simulink model "test_kinematics_sim"  (R2021b)
settings: Solver=ode8  StartTime=0.0  StopTime=100  FixedStep=0.01  RelTol=1e-3
values from neighbouring files (symbols this model uses):
  A = A0t'    [test_kinematics.m]
  e_angles0 = [atan(-A(2,1)/A(2,2)),asin(A(2,3)),atan(-A(1,3)/A(3,3))]    [test_kinematics.m]
  h0 = [Ix*omega0(1) Iy*omega0(2) Iz*omega0(3)]'    [test_kinematics.m]
  invJ = inv(J)    [test_kinematics.m]
  J = [Ix 0 0; 0 Iy 0; 0 0 Iz]    [test_kinematics.m]
  omega0 = [C 0.1 0.1]    [test_kinematics.m]
libraries: kinematic_transform x1, kinematics x1
settings Model: Creator=Davide  LastModifiedBy=Davide

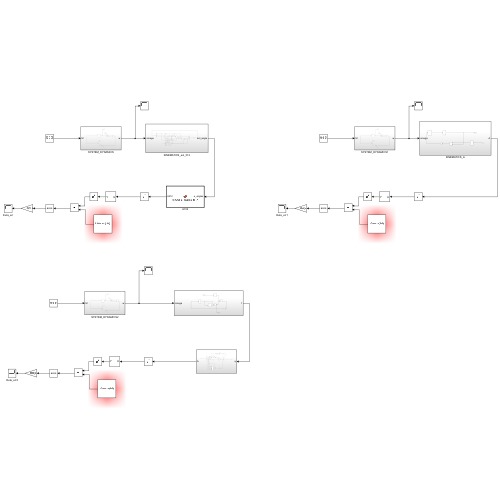
[thumbnail: Simulink's stored preview of the top-level diagram]
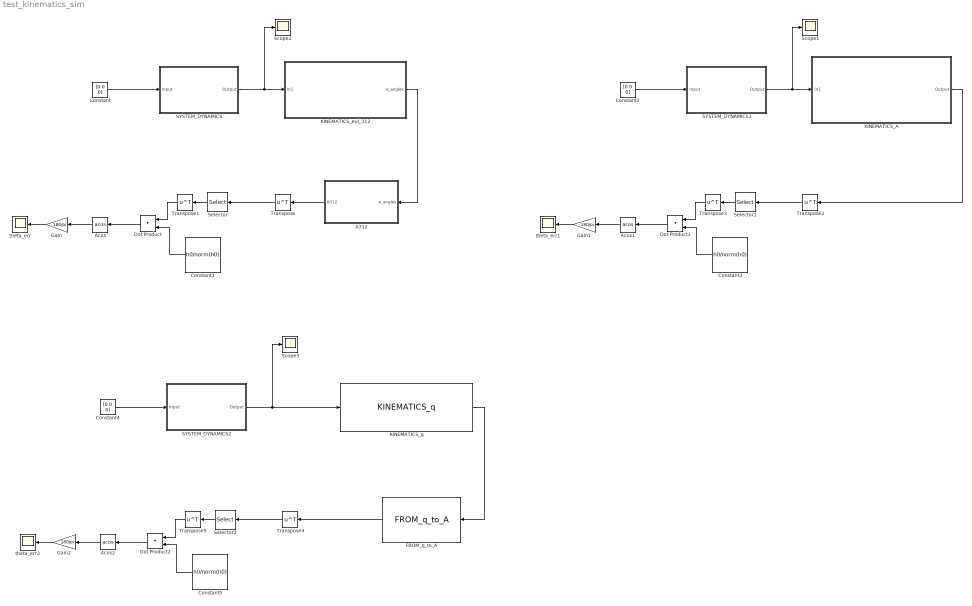
== system test_kinematics_sim ==
  A312 : MATLAB Function  TreatAsAtomicUnit=on
  Acos : Trigonometry  Operator=acos
  Acos1 : Trigonometry  Operator=acos
  Acos2 : Trigonometry  Operator=acos
  Constant : Constant  Value=[0 0 0]
  Constant1 : Constant  Value=h0/norm(h0)
  Constant2 : Constant  Value=[0 0 0]
  Constant3 : Constant  Value=h0/norm(h0)
  Constant4 : Constant  Value=[0 0 0]
  Constant5 : Constant  Value=h0/norm(h0)
  Dot Product : DotProduct  InputSameDT=on  OutDataTypeStr=Inherit: Inherit via internal rule
  Dot Product1 : DotProduct  InputSameDT=on  OutDataTypeStr=Inherit: Inherit via internal rule
  Dot Product2 : DotProduct  InputSameDT=on  OutDataTypeStr=Inherit: Inherit via internal rule
  FROM_q_to_A : kinematic_transform/FROM_q_to_A  SystemSampleTime=-1  VariantActivationTime=update diagram  Latency=0  AutoFrameSizeCalculation=off
      settings: SourceProductName=Kinematic Tranformation
  Gain : Gain  Gain=180/pi
  Gain1 : Gain  Gain=180/pi
  Gain2 : Gain  Gain=180/pi
  KINEMATICS_A : Subsystem
  KINEMATICS_eul_312 : Subsystem
  KINEMATICS_q : kinematics/KINEMATICS_q  SystemSampleTime=-1  VariantActivationTime=update diagram  Latency=0  AutoFrameSizeCalculation=off
  SYSTEM_DYNAMICS : Subsystem
  SYSTEM_DYNAMICS1 : Subsystem
  SYSTEM_DYNAMICS2 : Subsystem
  Scope1 : Scope
  Scope2 : Scope
  Scope3 : Scope
  Selector : Selector  NumberOfDimensions=2  InputPortWidth=3  IndexOptions=Index vector (dialog),Select all  Indices=1,1  OutputSizes=1,1
  Selector1 : Selector  NumberOfDimensions=2  InputPortWidth=3  IndexOptions=Index vector (dialog),Select all  Indices=1,1  OutputSizes=1,1
  Selector2 : Selector  NumberOfDimensions=2  InputPortWidth=3  IndexOptions=Index vector (dialog),Select all  Indices=1,1  OutputSizes=1,1
  Transpose{,1..5} (6 alike) : Math  Operator=transpose  SaturateOnIntegerOverflow=on
  theta_err : Scope
  theta_err1 : Scope
  theta_err2 : Scope
  wires:
  Constant/1 -> SYSTEM_DYNAMICS/1(Input)
  SYSTEM_DYNAMICS/1(Output) -> KINEMATICS_eul_312/1(In1), Scope2/1
  A312/1(A312) -> Transpose/1
  Selector/1 -> Transpose1/1
  Constant1/1 -> Dot Product/2
  Dot Product/1 -> Acos/1
  Acos/1 -> Gain/1
  Gain/1 -> theta_err/1
  Transpose1/1 -> Dot Product/1
  KINEMATICS_eul_312/1(e_angles) -> A312/1(e_angles)
  Transpose/1 -> Selector/1
  KINEMATICS_A/1(Output) -> Transpose2/1
  Gain1/1 -> theta_err1/1
  Transpose3/1 -> Dot Product1/1
  Selector1/1 -> Transpose3/1
  SYSTEM_DYNAMICS1/1(Output) -> KINEMATICS_A/1(In1), Scope1/1
  Acos1/1 -> Gain1/1
  Transpose2/1 -> Selector1/1
  Constant3/1 -> Dot Product1/2
  Dot Product1/1 -> Acos1/1
  Constant2/1 -> SYSTEM_DYNAMICS1/1(Input)
  Dot Product2/1 -> Acos2/1
  SYSTEM_DYNAMICS2/1(Output) -> Scope3/1, KINEMATICS_q/1
  Acos2/1 -> Gain2/1
  Constant4/1 -> SYSTEM_DYNAMICS2/1(Input)
  Selector2/1 -> Transpose5/1
  Transpose5/1 -> Dot Product2/1
  Gain2/1 -> theta_err2/1
  Transpose4/1 -> Selector2/1
  Constant5/1 -> Dot Product2/2
  FROM_q_to_A/1 -> Transpose4/1
  KINEMATICS_q/1 -> FROM_q_to_A/1

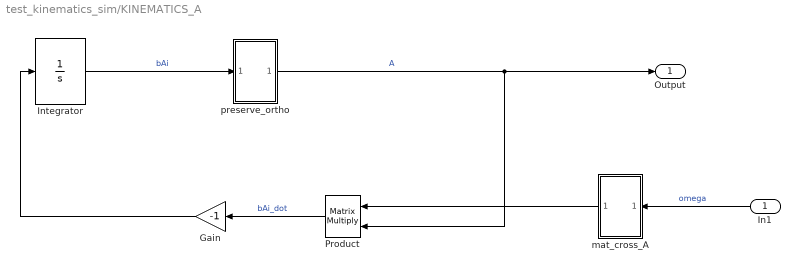
== system test_kinematics_sim/KINEMATICS_A ==
  In1 : Inport
  Gain : Gain  Gain=-1
  Integrator : Integrator  InitialCondition=A
  Product : Product  Multiplication=Matrix(*)
  mat_cross_A : Subsystem
  preserve_ortho : Subsystem
  Output : Outport
  wires:
  Integrator/1 -> preserve_ortho/1(In1)  "bAi"
  Product/1 -> Gain/1  "bAi_dot"
  In1/1 -> mat_cross_A/1(In1)  "omega"
  preserve_ortho/1(Out1) -> Output/1, Product/2  "A"
  mat_cross_A/1(Out1) -> Product/1
  Gain/1 -> Integrator/1

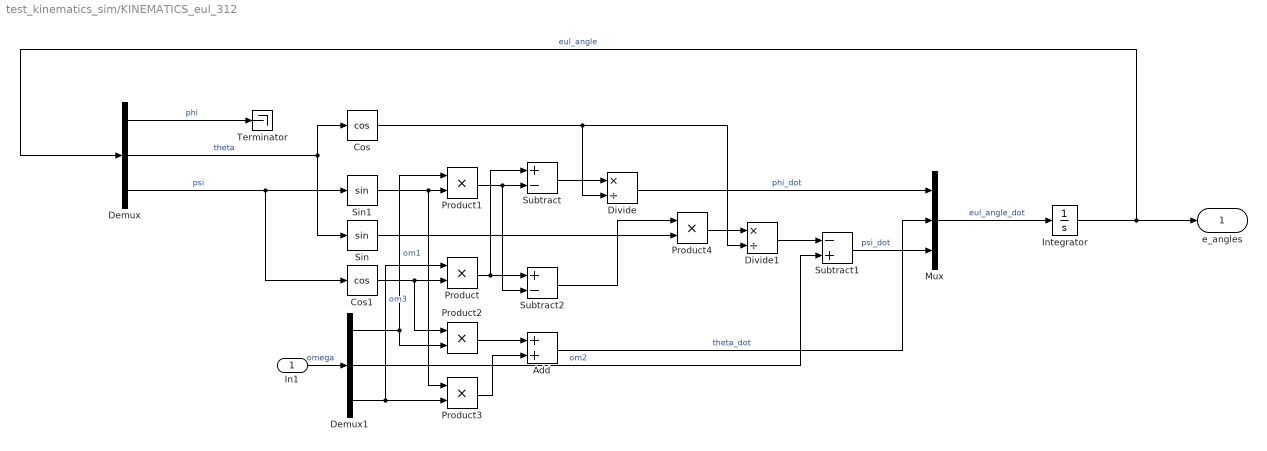
== system test_kinematics_sim/KINEMATICS_eul_312 ==
  In1 : Inport
  Add : Sum
  Cos : Trigonometry  Operator=cos
  Cos1 : Trigonometry  Operator=cos
  Demux : Demux  Outputs=3
  Demux1 : Demux  Outputs=3
  Divide : Product  Inputs=*/
  Divide1 : Product  Inputs=*/
  Integrator : Integrator  InitialCondition=e_angles0
  Mux : Mux  Inputs=3
  Product{,1..4} (5 alike) : Product
  Sin : Trigonometry
  Sin1 : Trigonometry
  Subtract : Sum  Inputs=+-
  Subtract1 : Sum  Inputs=-+
  Subtract2 : Sum  Inputs=+-
  Terminator : Terminator
  e_angles : Outport
  wires:
  Add/1 -> Mux/2  "theta_dot"
  In1/1 -> Demux1/1  "omega"
  Product2/1 -> Add/1
  Cos/1 -> Divide1/2, Divide/2
  Product3/1 -> Add/2
  Divide/1 -> Mux/1  "phi_dot"
  Demux/1 -> Terminator/1  "phi"
  Integrator/1 -> Demux/1, e_angles/1  "eul_angle"
  Cos1/1 -> Product2/1, Product/2
  Sin/1 -> Product4/2
  Product1/1 -> Subtract2/2, Subtract/2
  Divide1/1 -> Subtract1/1
  Demux/3 -> Sin1/1, Cos1/1  "psi"
  Subtract/1 -> Divide/1
  Demux1/3 -> Product3/2, Product/1  "om3"
  Mux/1 -> Integrator/1  "eul_angle_dot"
  Product/1 -> Subtract2/1, Subtract/1
  Product4/1 -> Divide1/1
  Demux1/1 -> Product2/2, Product1/1  "om1"
  Demux/2 -> Cos/1, Sin/1  "theta"
  Sin1/1 -> Product3/1, Product1/2
  Subtract2/1 -> Product4/1
  Demux1/2 -> Subtract1/2  "om2"
  Subtract1/1 -> Mux/3  "psi_dot"

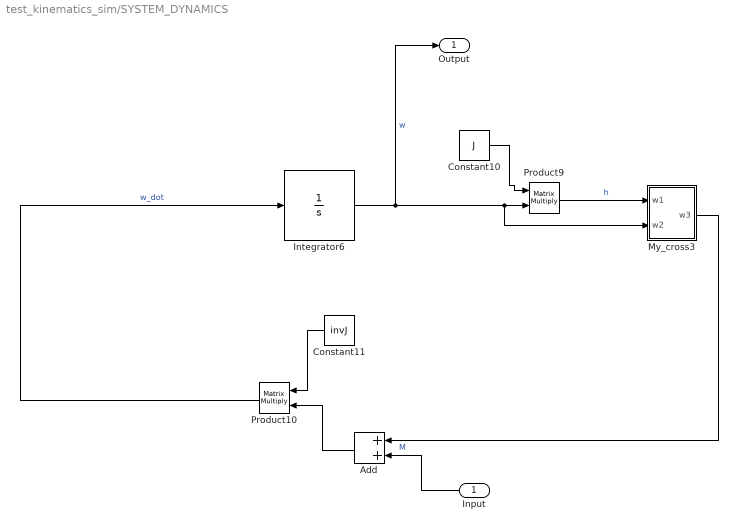
== system test_kinematics_sim/SYSTEM_DYNAMICS ==
  Input : Inport
  Add : Sum
  Constant10 : Constant  Value=J
  Constant11 : Constant  Value=invJ
  Integrator6 : Integrator  InitialCondition=omega0
  My_cross3 : Subsystem
  Product10 : Product  Multiplication=Matrix(*)
  Product9 : Product  Multiplication=Matrix(*)
  Output : Outport
  wires:
  Integrator6/1 -> Output/1, My_cross3/2(w2), Product9/2  "w"
  Constant10/1 -> Product9/1
  Constant11/1 -> Product10/1
  Product9/1 -> My_cross3/1(w1)  "h"
  My_cross3/1(w3) -> Add/1
  Product10/1 -> Integrator6/1  "w_dot"
  Input/1 -> Add/2  "M"
  Add/1 -> Product10/2

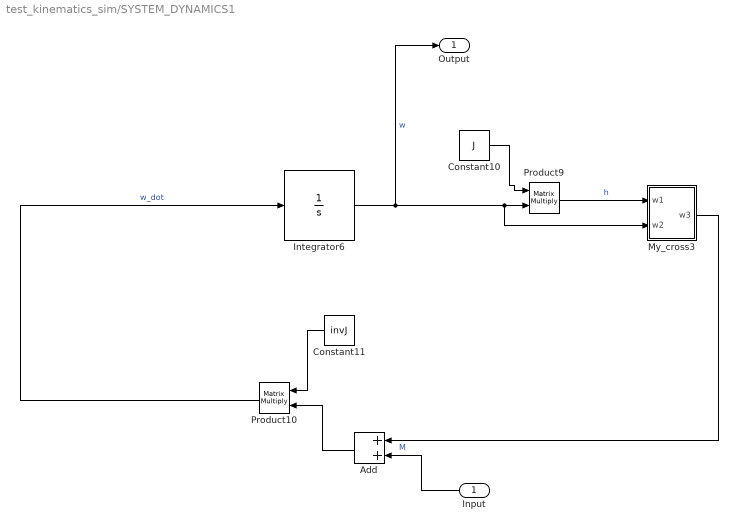
== system test_kinematics_sim/SYSTEM_DYNAMICS1 ==
  Input : Inport
  Add : Sum
  Constant10 : Constant  Value=J
  Constant11 : Constant  Value=invJ
  Integrator6 : Integrator  InitialCondition=omega0
  My_cross3 : Subsystem
  Product10 : Product  Multiplication=Matrix(*)
  Product9 : Product  Multiplication=Matrix(*)
  Output : Outport
  wires:
  Integrator6/1 -> Output/1, My_cross3/2(w2), Product9/2  "w"
  Constant10/1 -> Product9/1
  Constant11/1 -> Product10/1
  Product9/1 -> My_cross3/1(w1)  "h"
  My_cross3/1(w3) -> Add/1
  Product10/1 -> Integrator6/1  "w_dot"
  Input/1 -> Add/2  "M"
  Add/1 -> Product10/2

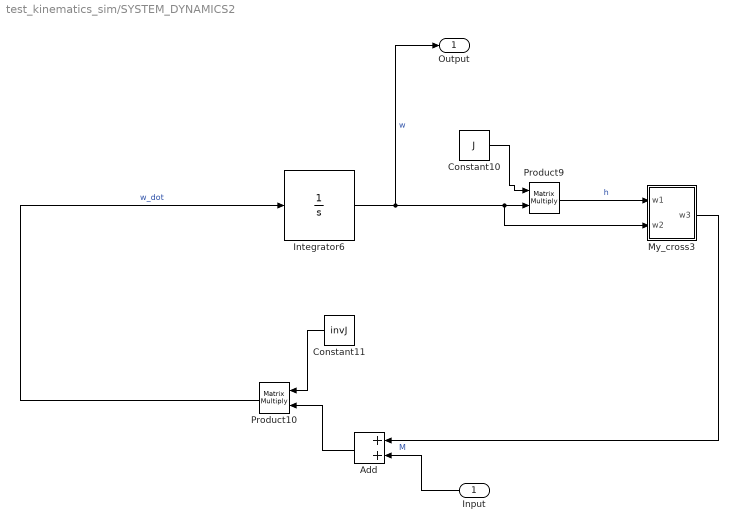
== system test_kinematics_sim/SYSTEM_DYNAMICS2 ==
  Input : Inport
  Add : Sum
  Constant10 : Constant  Value=J
  Constant11 : Constant  Value=invJ
  Integrator6 : Integrator  InitialCondition=omega0
  My_cross3 : Subsystem
  Product10 : Product  Multiplication=Matrix(*)
  Product9 : Product  Multiplication=Matrix(*)
  Output : Outport
  wires:
  Integrator6/1 -> Output/1, My_cross3/2(w2), Product9/2  "w"
  Constant10/1 -> Product9/1
  Constant11/1 -> Product10/1
  Product9/1 -> My_cross3/1(w1)  "h"
  My_cross3/1(w3) -> Add/1
  Product10/1 -> Integrator6/1  "w_dot"
  Input/1 -> Add/2  "M"
  Add/1 -> Product10/2

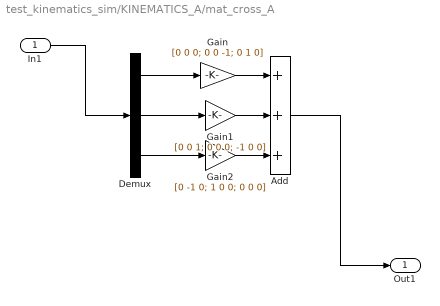
== system test_kinematics_sim/KINEMATICS_A/mat_cross_A ==
  In1 : Inport
  Add : Sum  Inputs=+++
  Demux : Demux  Outputs=3
  Gain : Gain  Gain=[0 0 0; 0 0 -1; 0 1 0]
  Gain1 : Gain  Gain=[0 0 1; 0 0 0; -1 0 0]
  Gain2 : Gain  Gain=[0 -1 0; 1 0 0; 0 0 0]
  Out1 : Outport
  wires:
  In1/1 -> Demux/1
  Gain1/1 -> Add/2
  Gain2/1 -> Add/3
  Demux/2 -> Gain1/1
  Add/1 -> Out1/1
  Gain/1 -> Add/1
  Demux/3 -> Gain2/1
  Demux/1 -> Gain/1

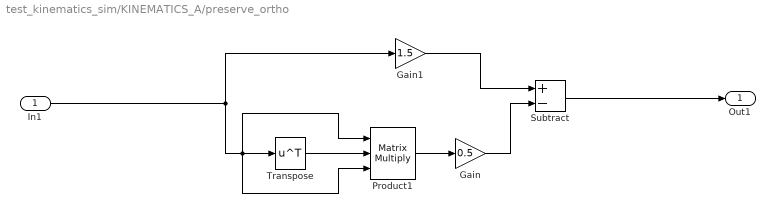
== system test_kinematics_sim/KINEMATICS_A/preserve_ortho ==
  In1 : Inport
  Gain : Gain  Gain=0.5
  Gain1 : Gain  Gain=1.5
  Product1 : Product  Inputs=3  Multiplication=Matrix(*)
  Subtract : Sum  Inputs=+-
  Transpose : Math  Operator=transpose  SaturateOnIntegerOverflow=on
  Out1 : Outport
  wires:
  In1/1 -> Product1/3, Product1/1, Transpose/1, Gain1/1
  Gain1/1 -> Subtract/1
  Product1/1 -> Gain/1
  Gain/1 -> Subtract/2
  Transpose/1 -> Product1/2
  Subtract/1 -> Out1/1

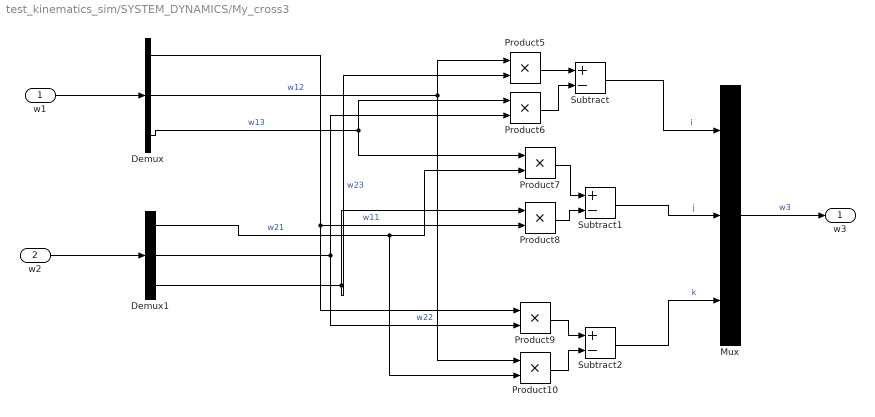
== system test_kinematics_sim/SYSTEM_DYNAMICS/My_cross3 ==
  w1 : Inport
  w2 : Inport  Port=2
  Demux : Demux  Outputs=3
  Demux1 : Demux  Outputs=3
  Mux : Mux  Inputs=3
  Product{5..10} (6 alike) : Product
  Subtract : Sum  Inputs=+-
  Subtract1 : Sum  Inputs=+-
  Subtract2 : Sum  Inputs=+-
  w3 : Outport
  wires:
  Subtract1/1 -> Mux/2  "j"
  Product6/1 -> Subtract/2
  Demux1/3 -> Product5/2, Product8/1  "w23"
  Demux/1 -> Product9/1, Product8/2  "w11"
  Demux/3 -> Product7/1, Product6/1  "w13"
  Product5/1 -> Subtract/1
  Demux1/1 -> Product10/2, Product7/2  "w21"
  Product9/1 -> Subtract2/1
  Demux1/2 -> Product9/2, Product6/2  "w22"
  Demux/2 -> Product5/1, Product10/1  "w12"
  Subtract/1 -> Mux/1  "i"
  w2/1 -> Demux1/1
  Product10/1 -> Subtract2/2
  Product7/1 -> Subtract1/1
  Product8/1 -> Subtract1/2
  Subtract2/1 -> Mux/3  "k"
  w1/1 -> Demux/1
  Mux/1 -> w3/1  "w3"

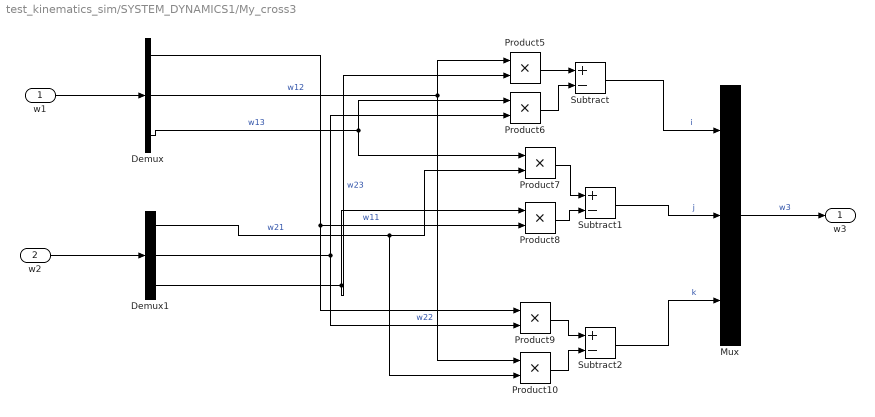
== system test_kinematics_sim/SYSTEM_DYNAMICS1/My_cross3 ==
  w1 : Inport
  w2 : Inport  Port=2
  Demux : Demux  Outputs=3
  Demux1 : Demux  Outputs=3
  Mux : Mux  Inputs=3
  Product{5..10} (6 alike) : Product
  Subtract : Sum  Inputs=+-
  Subtract1 : Sum  Inputs=+-
  Subtract2 : Sum  Inputs=+-
  w3 : Outport
  wires:
  Subtract1/1 -> Mux/2  "j"
  Product6/1 -> Subtract/2
  Demux1/3 -> Product5/2, Product8/1  "w23"
  Demux/1 -> Product9/1, Product8/2  "w11"
  Demux/3 -> Product7/1, Product6/1  "w13"
  Product5/1 -> Subtract/1
  Demux1/1 -> Product10/2, Product7/2  "w21"
  Product9/1 -> Subtract2/1
  Demux1/2 -> Product9/2, Product6/2  "w22"
  Demux/2 -> Product5/1, Product10/1  "w12"
  Subtract/1 -> Mux/1  "i"
  w2/1 -> Demux1/1
  Product10/1 -> Subtract2/2
  Product7/1 -> Subtract1/1
  Product8/1 -> Subtract1/2
  Subtract2/1 -> Mux/3  "k"
  w1/1 -> Demux/1
  Mux/1 -> w3/1  "w3"

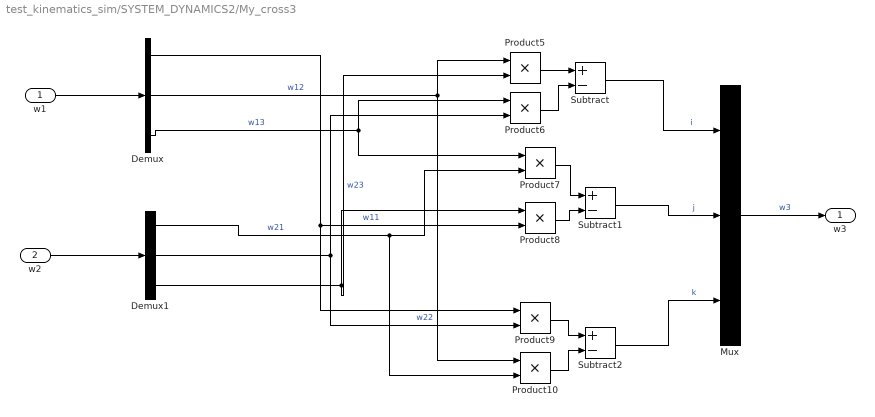
== system test_kinematics_sim/SYSTEM_DYNAMICS2/My_cross3 ==
  w1 : Inport
  w2 : Inport  Port=2
  Demux : Demux  Outputs=3
  Demux1 : Demux  Outputs=3
  Mux : Mux  Inputs=3
  Product{5..10} (6 alike) : Product
  Subtract : Sum  Inputs=+-
  Subtract1 : Sum  Inputs=+-
  Subtract2 : Sum  Inputs=+-
  w3 : Outport
  wires:
  Subtract1/1 -> Mux/2  "j"
  Product6/1 -> Subtract/2
  Demux1/3 -> Product5/2, Product8/1  "w23"
  Demux/1 -> Product9/1, Product8/2  "w11"
  Demux/3 -> Product7/1, Product6/1  "w13"
  Product5/1 -> Subtract/1
  Demux1/1 -> Product10/2, Product7/2  "w21"
  Product9/1 -> Subtract2/1
  Demux1/2 -> Product9/2, Product6/2  "w22"
  Demux/2 -> Product5/1, Product10/1  "w12"
  Subtract/1 -> Mux/1  "i"
  w2/1 -> Demux1/1
  Product10/1 -> Subtract2/2
  Product7/1 -> Subtract1/1
  Product8/1 -> Subtract1/2
  Subtract2/1 -> Mux/3  "k"
  w1/1 -> Demux/1
  Mux/1 -> w3/1  "w3"

== matlab function test_kinematics_sim/A312 ==
  data: e_angles input; A312 output
function A312 = FROM_e_angles_to_A(e_angles)
phi = e_angles(1);
theta = e_angles(2);
psi = e_angles(3);
A312 = [cos(psi)*cos(phi)-sin(psi)*sin(phi)*sin(theta), cos(psi)*sin(phi) + sin(psi)*cos(phi)*sin(theta), -sin(psi)*cos(theta);
     -sin(phi)*cos(theta), cos(phi)*cos(theta), sin(theta);
     sin(psi)*cos(phi)+cos(psi)*sin(phi)*sin(theta), sin(psi)*sin(phi)-cos(psi)*cos(phi)*sin(theta), cos(theta)*cos(psi)];
end
